simulink model "modelo_mecanico"  (R2016a)
settings: Solver=VariableStepAuto  StartTime=0.0  StopTime=10.0  RelTol=1e-3
settings Model: Creator=Pichau  LastModifiedBy=Pichau

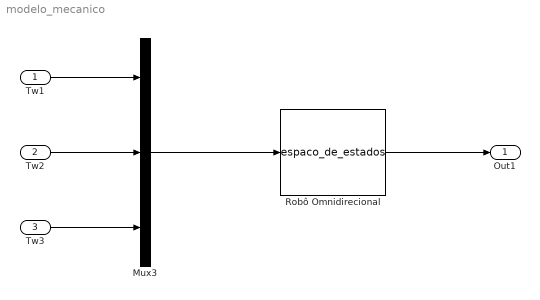
== system modelo_mecanico ==
  Tw1 : Inport
  Tw2 : Inport  Port=2
  Tw3 : Inport  Port=3
  Mux3 : Mux  Inputs=3
  Robô Omnidirecional : S-Function  FunctionName=espaco_de_estados  Parameters=r,m,Jw,J,L  SFunctionDeploymentMode=off  EnableBusSupport=off  mask{r=0.072, m=1.71, Jw=8.1e-4, J=2.125, L=0.09}
      mask prompts: r "r (m)"; m "m (Kg)"; Jw "Jw (Kg*m^2)"; J "J (Kg*m^2)"; L "L (m)"
      mask Display: image(imread('Robot_omnidirectional_drive.png'));
  Out1 : Outport
  wires:
  Mux3/1 -> Robô Omnidirecional/1
  Tw3/1 -> Mux3/3
  Tw2/1 -> Mux3/2
  Tw1/1 -> Mux3/1
  Robô Omnidirecional/1 -> Out1/1
